simulink model "SafetyCriticalLQRRobustCBF"  (R2020b)
settings: Solver=VariableStepAuto  StartTime=0.0  StopTime=tf_upperbound  RelTol=1e-7
PreLoadFcn:
  | SafetyCriticalLQRParams
values from neighbouring files (symbols this model uses):
  A = [0 0 0 0 0 0 0 0 1 0 0 0 ... (16 elements, 4x4)]    [RobustECBFDesign.mat]    (also in SafetyCriticalLQRParams.m = [     0 0 1 0;     0 0 0 1;     0 0 0 0;     0 0 0 0)
  B = [0  0; 0  0; 1  0; 0  1]    [RobustECBFDesign.mat]    (also in SafetyCriticalLQRParams.m = [0 0;0 0;1 0;0 1])
  beta = 0.6    [RobustECBFDesign.mat]    (also in SafetyCriticalLQRParams.m; hMATLABfcn.m = Input(1))
  C = [1 0 0 0 0 1 0 0 0 0 1 0 ... (16 elements, 4x4)]    [RobustECBFDesign.mat]    (also in SafetyCriticalLQRParams.m = eye(4))
  cT = [-2 -2.5]    [RobustECBFDesign.mat]    (also in SafetyCriticalLQRParams.m = [-2,-2.5]; hMATLABfcn.m = Input(2:3))
  D = [0  0; 0  0; 0  0; 0  0]    [RobustECBFDesign.mat]    (also in SafetyCriticalLQRParams.m = zeros(4,2))
  K = [1  1.26505863265e-16  3.46410161514  -2.97223693372e-18; 2.33155507841e-17  1  1.40474432322e-16  3.46410161514]    [RobustECBFDesign.mat]
  Ref = [0 0 0 0]    [RobustECBFDesign.mat]    (also in SafetyCriticalLQRParams.m = [0;0;0;0])
  rT = 1.5    [RobustECBFDesign.mat]    (also in SafetyCriticalLQRParams.m; hMATLABfcn.m = Input(4))
  x0 = [-5 -5 0 0]    [RobustECBFDesign.mat]    (also in SafetyCriticalLQRParams.m = [-5;-5;0;0])
libraries: simulink x1
settings Model: Creator=Jyot Buch  LastModifiedBy=Jyot Buch

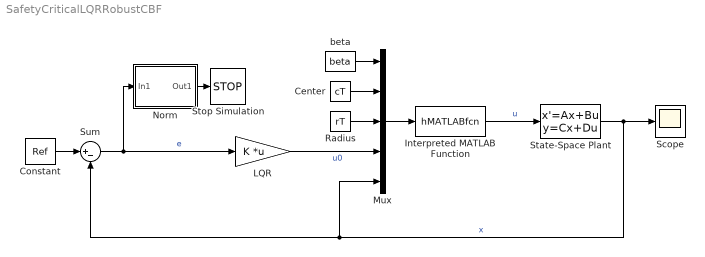
== system SafetyCriticalLQRRobustCBF ==
  Center : Constant  Value=cT
  Constant : Constant  Value=Ref
  Interpreted MATLAB Function : MATLABFcn  MATLABFcn=hMATLABfcn
  LQR : Gain  Gain=K  Multiplication=Matrix(K*u) (u vector)
  Mux : Mux  Inputs=5
  Norm : Subsystem
  Radius : Constant  Value=rT
  Scope : Scope
  State-Space Plant : StateSpace  A=A  B=B  C=C  D=D  InitialCondition=x0
  Stop Simulation : Stop
  Sum : Sum  Inputs=|+-
  beta : Constant  Value=beta
  wires:
  State-Space Plant/1 -> Mux/5, Sum/2, Scope/1  "x"
  Constant/1 -> Sum/1
  Sum/1 -> LQR/1, Norm/1(In1)  "e"
  Interpreted MATLAB Function/1 -> State-Space Plant/1  "u"
  beta/1 -> Mux/1
  Norm/1(Out1) -> Stop Simulation/1
  Mux/1 -> Interpreted MATLAB Function/1
  LQR/1 -> Mux/4  "u0"
  Radius/1 -> Mux/3
  Center/1 -> Mux/2

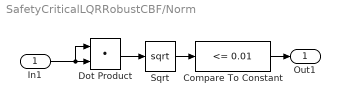
== system SafetyCriticalLQRRobustCBF/Norm ==
  In1 : Inport
  Compare To Constant : simulink/Logic and Bit Operations/Compare To Constant  relop=<=  const=0.01  OutDataTypeStr=boolean
  Dot Product : DotProduct  InputSameDT=on  OutDataTypeStr=Inherit: Inherit via internal rule
  Sqrt : Sqrt  SaturateOnIntegerOverflow=on
  Out1 : Outport
  wires:
  In1/1 -> Dot Product/1, Dot Product/2
  Dot Product/1 -> Sqrt/1
  Sqrt/1 -> Compare To Constant/1
  Compare To Constant/1 -> Out1/1
